simulink model "Commande_Simscape_ModelePhysique"  (R2015a)
settings: Solver=ode23t  StartTime=0.0  StopTime=10.0  RelTol=1e-3
InitFcn:
  | load('LeftInput_Measures.mat');
  | load('LeftOutput_Measures.mat');
  | Parametres_Rover
undefined symbols (not defined in the file): DL, DR, EncRes, IL, IR, NL, NR, PL, PR, r, RroueL, RroueR
libraries: SingleMotor_Duty_to_inc x4, SingleMotor_V_to_rads x2, simulink x2, MarsRover_SimMechanics x1
settings Model: Creator=tbaroche  LastModifiedBy=tbaroche

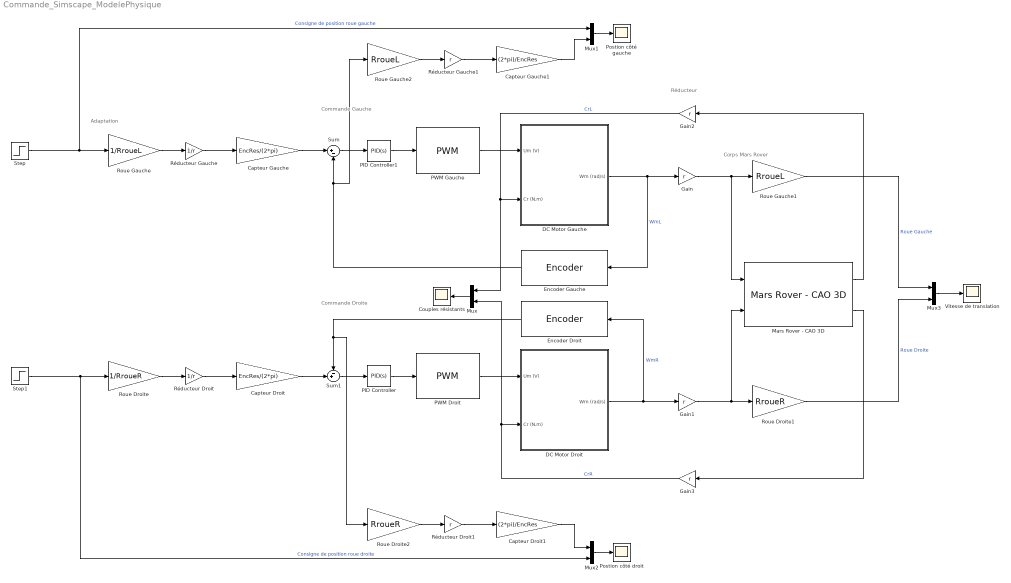
== system Commande_Simscape_ModelePhysique ==
  note: Adaptation
  note: Réducteur
  note: Commande Gauche
  note: Commande Droite
  note: Corps Mars Rover
  Capteur Droit : Gain  Gain=EncRes/(2*pi)
  Capteur Droit1 : Gain  Gain=(2*pi)/EncRes
  Capteur Gauche : Gain  Gain=EncRes/(2*pi)
  Capteur Gauche1 : Gain  Gain=(2*pi)/EncRes
  Couples résistants : Scope
      settings: YMin=-0.0015  YMax=0.003
  DC Motor Droit : Subsystem  BlockChoice=Modèle Simscape
      link override "SimElectronics Model ": Kphi_lib=Kphi  Rm_lib=Rm  Lm_lib=Lm  bm_lib=bm  Jm_lib=Jm
      link override SimElectronics Model /Simulink-PS Converter/input0: OutDataTypeStr=double  PortDimensions=-1
      link override SimElectronics Model /Simulink-PS Converter1/input0: OutDataTypeStr=double  PortDimensions=-1
      settings: AttributesFormatString=%<BlockChoice>  TemplateBlock=SingleMotor_V_to_rads/DC Motor  MemberBlocks=Modèle Simscape,Modèle Simulink
  DC Motor Gauche : Subsystem  BlockChoice=Modèle Simscape
      link override "SimElectronics Model ": Kphi_lib=Kphi  Rm_lib=Rm  Lm_lib=Lm  bm_lib=bm  Jm_lib=Jm
      settings: AttributesFormatString=%<BlockChoice>  TemplateBlock=SingleMotor_V_to_rads/DC Motor  MemberBlocks=Modèle Simscape,Modèle Simulink
  Encoder Droit : SingleMotor_Duty_to_inc/Encoder  EncRes=EncRes
  Encoder Gauche : SingleMotor_Duty_to_inc/Encoder  EncRes=EncRes
  Gain{,1..3} (4 alike) : Gain  Gain=r
  Mars Rover - CAO 3D : MarsRover_SimMechanics/Mars Rover - CAO 3D
  Mux{,1..3} (4 alike) : Mux  Inputs=2
  PID Controller : simulink/Continuous/PID Controller  Controller=PID  TimeDomain=Continuous-time  SampleTime=-1  IntegratorMethod=Forward Euler  FilterMethod=Forward Euler  Form=Parallel  UseFilter=on  ControllerParametersSource=internal  P=PR  I=IR  D=DR  N=NR  InitialConditionSource=internal  InitialConditionForIntegrator=0  InitialConditionForFilter=0  ExternalReset=none  LimitOutput=off  UpperSaturationLimit=inf  LowerSaturationLimit=-inf  LinearizeAsGain=on  AntiWindupMode=none  Kb=1  TrackingMode=off  Kt=1  PParamMin=[]  PParamMax=[]  IParamMin=[]  IParamMax=[]  DParamMin=[]  DParamMax=[]  NParamMin=[]  NParamMax=[]  KbParamMin=[]  KbParamMax=[]  KtParamMin=[]  KtParamMax=[]  POutMin=[]  POutMax=[]  IOutMin=[]  IOutMax=[]  DOutMin=[]  DOutMax=[]  NOutMin=[]  NOutMax=[]  KbOutMin=[]  KbOutMax=[]  KtOutMin=[]  KtOutMax=[]  IntegratorOutMin=[]  IntegratorOutMax=[]  FilterOutMin=[]  FilterOutMax=[]  SumOutMin=[]  SumOutMax=[]  SumI1OutMin=[]  SumI1OutMax=[]  SumI2OutMin=[]  SumI2OutMax=[]  SumI3OutMin=[]  SumI3OutMax=[]  SumDOutMin=[]  SumDOutMax=[]  SaturationOutMin=[]  SaturationOutMax=[]  IntegratorContinuousStateAttributes=''  IntegratorStateMustResolveToSignalObject=off  IntegratorRTWStateStorageClass=Auto  FilterContinuousStateAttributes=''  FilterStateMustResolveToSignalObject=off  FilterRTWStateStorageClass=Auto  DifferentiatorICPrevScaledInput=0  DifferentiatorOutMin=[]  DifferentiatorOutMax=[]
  PID Controller1 : simulink/Continuous/PID Controller  Controller=PID  TimeDomain=Continuous-time  SampleTime=-1  IntegratorMethod=Forward Euler  FilterMethod=Forward Euler  Form=Parallel  UseFilter=on  ControllerParametersSource=internal  P=PL  I=IL  D=DL  N=NL  InitialConditionSource=internal  InitialConditionForIntegrator=0  InitialConditionForFilter=0  ExternalReset=none  LimitOutput=off  UpperSaturationLimit=inf  LowerSaturationLimit=-inf  LinearizeAsGain=on  AntiWindupMode=none  Kb=1  TrackingMode=off  Kt=1  PParamMin=[]  PParamMax=[]  IParamMin=[]  IParamMax=[]  DParamMin=[]  DParamMax=[]  NParamMin=[]  NParamMax=[]  KbParamMin=[]  KbParamMax=[]  KtParamMin=[]  KtParamMax=[]  POutMin=[]  POutMax=[]  IOutMin=[]  IOutMax=[]  DOutMin=[]  DOutMax=[]  NOutMin=[]  NOutMax=[]  KbOutMin=[]  KbOutMax=[]  KtOutMin=[]  KtOutMax=[]  IntegratorOutMin=[]  IntegratorOutMax=[]  FilterOutMin=[]  FilterOutMax=[]  SumOutMin=[]  SumOutMax=[]  SumI1OutMin=[]  SumI1OutMax=[]  SumI2OutMin=[]  SumI2OutMax=[]  SumI3OutMin=[]  SumI3OutMax=[]  SumDOutMin=[]  SumDOutMax=[]  SaturationOutMin=[]  SaturationOutMax=[]  IntegratorContinuousStateAttributes=''  IntegratorStateMustResolveToSignalObject=off  IntegratorRTWStateStorageClass=Auto  FilterContinuousStateAttributes=''  FilterStateMustResolveToSignalObject=off  FilterRTWStateStorageClass=Auto  DifferentiatorICPrevScaledInput=0  DifferentiatorOutMin=[]  DifferentiatorOutMax=[]
  PWM Droit : SingleMotor_Duty_to_inc/PWM  FreqTriangle=FreqPWM
  PWM Gauche : SingleMotor_Duty_to_inc/PWM  FreqTriangle=FreqPWM
  Postion côté droit : Scope
      settings: YMin=-0.0015  YMax=0.003  SaveName=ScopeData2
  Postion côté gauche : Scope
      settings: YMin=-0.0015  YMax=0.003
  Roue Droite : Gain  Gain=1/RroueR
  Roue Droite1 : Gain  Gain=RroueR
  Roue Droite2 : Gain  Gain=RroueR
  Roue Gauche : Gain  Gain=1/RroueL
  Roue Gauche1 : Gain  Gain=RroueL
  Roue Gauche2 : Gain  Gain=RroueL
  Réducteur Droit : Gain  Gain=1/r
  Réducteur Droit1 : Gain  Gain=r
  Réducteur Gauche : Gain  Gain=1/r
  Réducteur Gauche1 : Gain  Gain=r
  Step : Step  Time=3  After=0.010  SampleTime=0
  Step1 : Step  Time=3  After=0.010  SampleTime=0
  Sum : Sum  Inputs=|+-
  Sum1 : Sum  Inputs=-+|
  Vitesse de translation : Scope
      settings: YMin=5.55112e-17  YMax=1.8  SaveName=ScopeData3
  wires:
  PWM Droit/1 -> DC Motor Droit/1(Um (V))
  PWM Gauche/1 -> DC Motor Gauche/1(Um (V))
  Gain2/1 -> Mux/1, DC Motor Gauche/2(Cr (N.m))  "CrL"
  Gain/1 -> Roue Gauche1/1, Mars Rover - CAO 3D/1
  Gain1/1 -> Roue Droite1/1, Mars Rover - CAO 3D/2
  Gain3/1 -> DC Motor Droit/2(Cr (N.m)), Mux/2  "CrR"
  Mars Rover - CAO 3D/1 -> Gain2/1
  DC Motor Gauche/1(Wm (rad/s)) -> Encoder Gauche/1, Gain/1  "WmL"
  Mars Rover - CAO 3D/2 -> Gain3/1
  DC Motor Droit/1(Wm (rad/s)) -> Encoder Droit/1, Gain1/1  "WmR"
  Mux/1 -> Couples résistants/1
  Encoder Gauche/1 -> Roue Gauche2/1, Sum/2
  Sum/1 -> PID Controller1/1
  PID Controller1/1 -> PWM Gauche/1
  Sum1/1 -> PID Controller/1
  PID Controller/1 -> PWM Droit/1
  Step/1 -> Mux1/1, Roue Gauche/1  "Consigne de position roue gauche"
  Step1/1 -> Mux2/2, Roue Droite/1  "Consigne de position roue droite"
  Capteur Gauche/1 -> Sum/1
  Capteur Droit/1 -> Sum1/2
  Réducteur Droit/1 -> Capteur Droit/1
  Réducteur Gauche/1 -> Capteur Gauche/1
  Roue Gauche/1 -> Réducteur Gauche/1
  Roue Droite/1 -> Réducteur Droit/1
  Mux1/1 -> Postion côté gauche/1
  Encoder Droit/1 -> Roue Droite2/1, Sum1/1
  Roue Gauche1/1 -> Mux3/1  "Roue Gauche"
  Réducteur Gauche1/1 -> Capteur Gauche1/1
  Roue Gauche2/1 -> Réducteur Gauche1/1
  Capteur Gauche1/1 -> Mux1/2
  Mux3/1 -> Vitesse de translation/1
  Roue Droite1/1 -> Mux3/2  "Roue Droite"
  Mux2/1 -> Postion côté droit/1
  Réducteur Droit1/1 -> Capteur Droit1/1
  Roue Droite2/1 -> Réducteur Droit1/1
  Capteur Droit1/1 -> Mux2/1

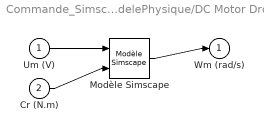
== system Commande_Simscape_ModelePhysique/DC Motor Droit ==
  Um (V) : Inport
  Cr (N.m) : Inport  Port=2
  Modèle Simscape : SingleMotor_V_to_rads/Modèle Simscape  Kphi_lib=Kphi  Rm_lib=Rm  Lm_lib=Lm  bm_lib=bm  Jm_lib=Jm
  Wm (rad/s) : Outport
  wires:
  Um (V)/1 -> Modèle Simscape/1
  Cr (N.m)/1 -> Modèle Simscape/2
  Modèle Simscape/1 -> Wm (rad/s)/1

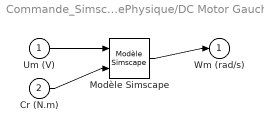
== system Commande_Simscape_ModelePhysique/DC Motor Gauche ==
  Um (V) : Inport
  Cr (N.m) : Inport  Port=2
  Modèle Simscape : SingleMotor_V_to_rads/Modèle Simscape  Kphi_lib=Kphi  Rm_lib=Rm  Lm_lib=Lm  bm_lib=bm  Jm_lib=Jm
  Wm (rad/s) : Outport
  wires:
  Um (V)/1 -> Modèle Simscape/1
  Cr (N.m)/1 -> Modèle Simscape/2
  Modèle Simscape/1 -> Wm (rad/s)/1
